simulink model "hdd_notch_final_3"  (R2015b)
settings: Solver=VariableStepAuto  StartTime=0.0  StopTime=1.1  RelTol=1e-3
undefined symbols (not defined in the file or in its folder): DiscIntNeverNeededParam
settings Model: disc_configurable_lib=simulink_discrete_with_notch_disc_lib  Creator=mac  LastModifiedBy=mac

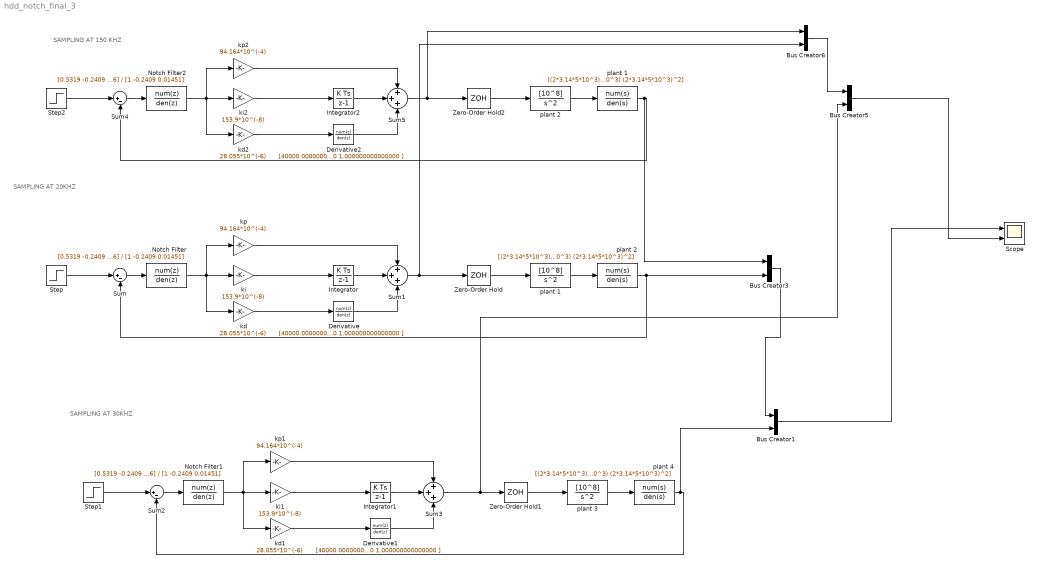
== system hdd_notch_final_3 ==
  note: SAMPLING AT 150 KHZ
  note: SAMPLING AT 20KHZ
  note: SAMPLING AT 30KHZ
  " plant 1" : TransferFcn  Numerator=[10^8]  Denominator=[1 0 0]
  " plant 2" : TransferFcn  Numerator=[10^8]  Denominator=[1 0 0]
  " plant 3" : TransferFcn  Numerator=[10^8]  Denominator=[1 0 0]
  Bus Creator{1,3,5..6} (4 alike) : BusCreator  Inputs=2
  Derivative : DiscreteTransferFcn  Numerator=[40000.000000000000000 -40000.000000000000000 ]  Denominator=[1.000000000000000 1.000000000000000 ]  SampleTime=6.67e-06
  Derivative1 : DiscreteTransferFcn  Numerator=[40000.000000000000000 -40000.000000000000000 ]  Denominator=[1.000000000000000 1.000000000000000 ]  SampleTime=2.5e-05
  Derivative2 : DiscreteTransferFcn  Numerator=[40000.000000000000000 -40000.000000000000000 ]  Denominator=[1.000000000000000 1.000000000000000 ]  SampleTime=5.55e-05
  Integrator : DiscreteIntegrator  SampleTime=6.67e-06  ICPrevOutput=DiscIntNeverNeededParam  ICPrevScaledInput=DiscIntNeverNeededParam  mask(DiscretizedDiscreteIntegrator){}
      mask init:
      | %zoh
  Integrator1 : DiscreteIntegrator  SampleTime=2.5e-05  ICPrevOutput=DiscIntNeverNeededParam  ICPrevScaledInput=DiscIntNeverNeededParam  mask(DiscretizedDiscreteIntegrator){}
      mask init:
      | %zoh
  Integrator2 : DiscreteIntegrator  SampleTime=5.55e-05  ICPrevOutput=DiscIntNeverNeededParam  ICPrevScaledInput=DiscIntNeverNeededParam  mask(DiscretizedDiscreteIntegrator){}
      mask init:
      | %zoh
  Notch Filter : DiscreteTransferFcn  Numerator=[0.5319 -0.2409 0.4826]  Denominator=[1 -0.2409 0.01451]  SampleTime=6.67e-06
  Notch Filter1 : DiscreteTransferFcn  Numerator=[0.5319 -0.2409 0.4826]  Denominator=[1 -0.2409 0.01451]  SampleTime=2.5e-05
  Notch Filter2 : DiscreteTransferFcn  Numerator=[0.5319 -0.2409 0.4826]  Denominator=[1 -0.2409 0.01451]  SampleTime=5.55e-05
  Scope : Scope  NumInputPorts=2
  Step : Step  SampleTime=5.00000000000000024e-05  mask(DiscretizedSource){}
      mask init:
      | %zoh
  Step1 : Step  SampleTime=2.5e-05  mask(DiscretizedSource){}
      mask init:
      | %zoh
  Step2 : Step  SampleTime=5.55e-05  mask(DiscretizedSource){}
      mask init:
      | %zoh
  Sum : Sum  Inputs=|+-
  Sum1 : Sum  Inputs=+++
  Sum2 : Sum  Inputs=|+-
  Sum3 : Sum  Inputs=+++
  Sum4 : Sum  Inputs=|+-
  Sum5 : Sum  Inputs=+++
  Zero-Order Hold : ZeroOrderHold  SampleTime=6.67e-06
  Zero-Order Hold1 : ZeroOrderHold  SampleTime=2.5e-05
  Zero-Order Hold2 : ZeroOrderHold  SampleTime=5.55e-05
  kd : Gain  Gain=28.055*10^(-6)
  kd1 : Gain  Gain=28.055*10^(-6)
  kd2 : Gain  Gain=28.055*10^(-6)
  ki : Gain  Gain=153.9*10^(-8)
  ki1 : Gain  Gain=153.9*10^(-8)
  ki2 : Gain  Gain=153.9*10^(-8)
  kp : Gain  Gain=94.164*10^(-4)
  kp1 : Gain  Gain=94.164*10^(-4)
  kp2 : Gain  Gain=94.164*10^(-4)
  plant 1 : TransferFcn  Numerator=[(2*3.14*5*10^3)^2]  Denominator="[1  2*0.05*(2*3.14*5*10^3) (2*3.14*5*10^3)^2]"
  plant 2 : TransferFcn  Numerator=[(2*3.14*5*10^3)^2]  Denominator="[1  2*0.05*(2*3.14*5*10^3) (2*3.14*5*10^3)^2]"
  plant 4 : TransferFcn  Numerator=[(2*3.14*5*10^3)^2]  Denominator="[1  2*0.05*(2*3.14*5*10^3) (2*3.14*5*10^3)^2]"
  wires:
  Zero-Order Hold/1 -> " plant 1"/1
  Sum1/1 -> Bus Creator6/2, Zero-Order Hold/1
  Integrator/1 -> Sum1/2
  ki/1 -> Integrator/1
  kd/1 -> Derivative/1
  Derivative/1 -> Sum1/3
  kp/1 -> Sum1/1
  Sum/1 -> Notch Filter/1
  Notch Filter/1 -> kp/1, kd/1, ki/1
  Step/1 -> Sum/1
  " plant 1"/1 -> plant 2/1
  plant 2/1 -> Bus Creator3/2, Sum/2
  Zero-Order Hold1/1 -> " plant 3"/1
  Sum3/1 -> Bus Creator5/2, Zero-Order Hold1/1
  Integrator1/1 -> Sum3/2
  ki1/1 -> Integrator1/1
  kd1/1 -> Derivative1/1
  Derivative1/1 -> Sum3/3
  kp1/1 -> Sum3/1
  Sum2/1 -> Notch Filter1/1
  Notch Filter1/1 -> kp1/1, kd1/1, ki1/1
  " plant 3"/1 -> plant 4/1
  plant 4/1 -> Bus Creator1/2, Sum2/2
  Step1/1 -> Sum2/1
  Zero-Order Hold2/1 -> " plant 2"/1
  Integrator2/1 -> Sum5/2
  ki2/1 -> Integrator2/1
  kd2/1 -> Derivative2/1
  Derivative2/1 -> Sum5/3
  kp2/1 -> Sum5/1
  Sum4/1 -> Notch Filter2/1
  Notch Filter2/1 -> kp2/1, kd2/1, ki2/1
  " plant 2"/1 -> plant 1/1
  plant 1/1 -> Bus Creator3/1, Sum4/2
  Step2/1 -> Sum4/1
  Sum5/1 -> Bus Creator6/1, Zero-Order Hold2/1
  Bus Creator6/1 -> Bus Creator5/1
  Bus Creator3/1 -> Bus Creator1/1
  Bus Creator1/1 -> Scope/1
  Bus Creator5/1 -> Scope/2
